simulink model "ejercicio1"  (R2022b)
settings: Solver=VariableStepAuto  StartTime=0.0  StopTime=10.0  RelTol=1e-3
settings Model: Creator=julianhinojosagil  LastModifiedBy=julianhinojosagil

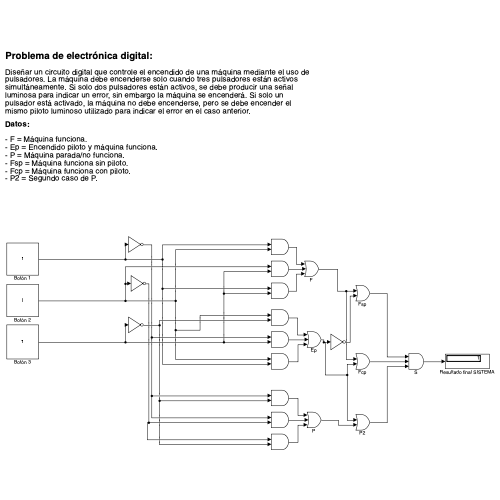
[thumbnail: Simulink's stored preview of the top-level diagram]
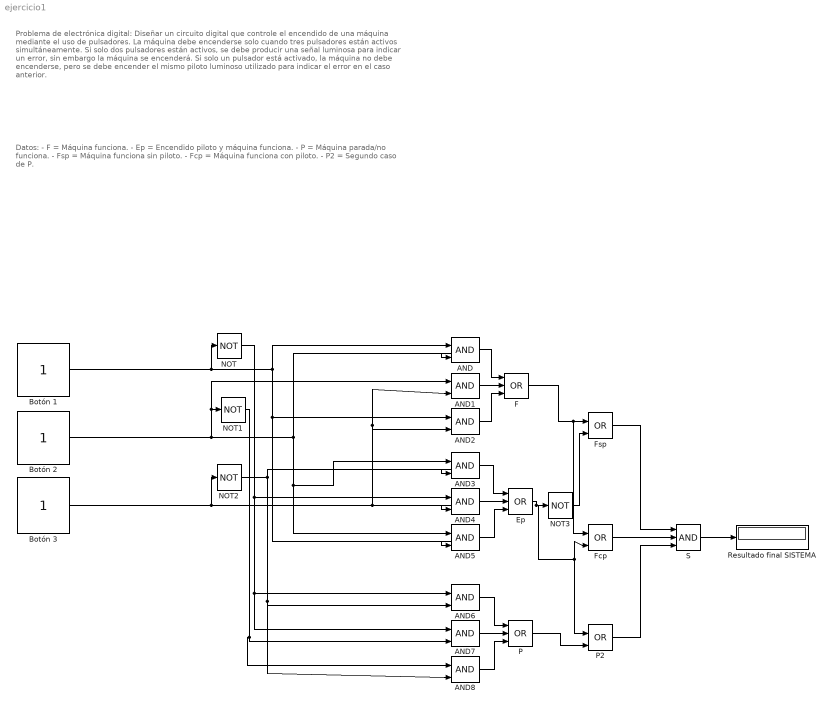
== system ejercicio1 ==
  note: Problema de electrónica digital:
      |
      | Diseñar un circuito digital que controle el encendido de una máquina mediante el uso de pulsadores. La máquina debe encenderse solo cuando tres pulsadores están activos simultáneamente. Si solo dos pulsadores están activos, se debe producir una señal luminosa para indicar un error, sin embargo la máquina se encenderá. Si solo un pulsador está activado, la máquina no debe encenderse, pero se debe encender el mismo piloto luminoso utilizado para indicar el error en el caso anterior.
  note: Datos:
      |
      | - F = Máquina funciona.
      | - Ep = Encendido piloto y máquina funciona.
      | - P = Máquina parada/no funciona.
      | - Fsp = Máquina funciona sin piloto.
      | - Fcp = Máquina funciona con piloto.
      | - P2 = Segundo caso de P.
  AND{,1..8} (9 alike) : Logic  IconShape=distinctive  AllPortsSameDT=off  OutDataTypeStr=boolean
  Botón 1 : Constant
  Botón 2 : Constant
  Botón 3 : Constant
  Ep : Logic  Operator=OR  Inputs=3  IconShape=distinctive  AllPortsSameDT=off  OutDataTypeStr=boolean
  F : Logic  Operator=OR  Inputs=3  IconShape=distinctive  AllPortsSameDT=off  OutDataTypeStr=boolean
  Fcp : Logic  Operator=OR  IconShape=distinctive  AllPortsSameDT=off  OutDataTypeStr=boolean
  Fsp : Logic  Operator=OR  IconShape=distinctive  AllPortsSameDT=off  OutDataTypeStr=boolean
  NOT{,1..3} (4 alike) : Logic  Operator=NOT  IconShape=distinctive  AllPortsSameDT=off  OutDataTypeStr=boolean
  P : Logic  Operator=OR  Inputs=3  IconShape=distinctive  AllPortsSameDT=off  OutDataTypeStr=boolean
  P2 : Logic  Operator=OR  IconShape=distinctive  AllPortsSameDT=off  OutDataTypeStr=boolean
  Resultado final SISTEMA : Display
  S : Logic  Inputs=3  IconShape=distinctive  AllPortsSameDT=off  OutDataTypeStr=boolean
  wires:
  Botón 1/1 -> NOT/1, AND5/2, AND2/1, AND/1
  Botón 2/1 -> AND1/1, NOT1/1, AND5/1, AND3/1, AND/2
  Botón 3/1 -> NOT2/1, AND4/2, AND2/2, AND1/2
  AND/1 -> F/1
  AND1/1 -> F/2
  AND2/1 -> F/3
  NOT2/1 -> AND8/2, AND6/2, AND3/2
  NOT/1 -> AND7/1, AND6/1, AND4/1
  AND3/1 -> Ep/1
  AND4/1 -> Ep/2
  AND5/1 -> Ep/3
  AND8/1 -> P/3
  AND7/1 -> P/2
  AND6/1 -> P/1
  NOT1/1 -> AND8/1, AND7/2
  Ep/1 -> Fcp/2, P2/1, NOT3/1
  F/1 -> Fcp/1, Fsp/1
  NOT3/1 -> Fsp/2
  P/1 -> P2/2
  Fsp/1 -> S/1
  Fcp/1 -> S/2
  P2/1 -> S/3
  S/1 -> Resultado final SISTEMA/1
